simulink model "F15_NDI"  (R2020b)
settings: Solver=ode4  StartTime=0.0  StopTime=10  FixedStep=0.01  RelTol=1e-3
libraries: pid_lib x6
settings Model: Creator=chenglingquan  LastModifiedBy=chenglingquan

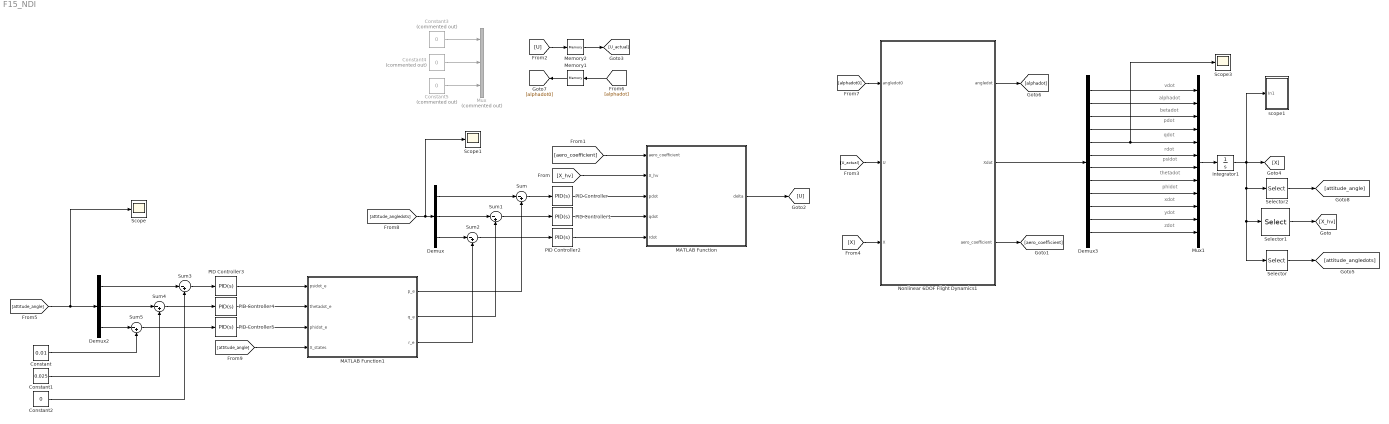
== system F15_NDI ==
  note: qdot
  note: thetadot
  note: zdot
  note: pdot
  note: ydot
  note: phidot
  note: xdot
  note: alphadot
  note: betadot
  note: psidot
  note: rdot
  note: vdot
  Constant : Constant  Value=0.01
  Constant1 : Constant  Value=0.025
  Constant2 : Constant  Value=0
  Constant3 : Constant  Commented=on  Value=0
  Constant4 : Constant  Commented=on  Value=0
  Constant5 : Constant  Commented=on  Value=0
  Demux : Demux  Outputs=3
  Demux2 : Demux  Outputs=3
  Demux3 : Demux  Outputs=12
  Integrator1 : Integrator  InitialCondition=[700,0.05,0,0,0,0,0,0,0,0,0,-6000]
  MATLAB Function : MATLAB Function  TreatAsAtomicUnit=on
  MATLAB Function1 : MATLAB Function  TreatAsAtomicUnit=on
  Memory1 : Memory  InitialCondition=[0,0]
  Memory2 : Memory  InitialCondition=[0,0,0]
  Mux : Mux  Commented=on  Inputs=3
  Mux1 : Mux  Inputs=12
  Nonlinear 6DOF Flight Dynamics1 : MATLAB Function  TreatAsAtomicUnit=on
  PID Controller : pid_lib/PID Controller  Controller=PID  Form=Parallel  TimeDomain=Continuous-time  UseExternalTs=off  SampleTime=-1  IntegratorMethod=Forward Euler  FilterMethod=Forward Euler  ControllerParametersSource=internal  P=50  I=1000  D=0  UseFilter=on  N=10000  TunerSelectOption=Transfer Function Based (PID Tuner App)  InitialConditionSource=internal  InitialConditionForIntegrator=0  InitialConditionForFilter=0  DifferentiatorICPrevScaledInput=0  ExternalReset=none  TrackingMode=off  Kt=1  LimitOutput=off  SatLimitsSource=internal  UpperSaturationLimit=inf  LowerSaturationLimit=-inf  LinearizeAsGain=on  AntiWindupMode=none  Kb=1  POutMin=[]  POutMax=[]  IOutMin=[]  IOutMax=[]  DOutMin=[]  DOutMax=[]  NOutMin=[]  NOutMax=[]  SumOutMin=[]  SumOutMax=[]  SaturationOutMin=[]  SaturationOutMax=[]  PParamMin=[]  PParamMax=[]  IParamMin=[]  IParamMax=[]  DParamMin=[]  DParamMax=[]  NParamMin=[]  NParamMax=[]  KbParamMin=[]  KbParamMax=[]  KtParamMin=[]  KtParamMax=[]  KbOutMin=[]  KbOutMax=[]  KtOutMin=[]  KtOutMax=[]  IntegratorOutMin=[]  IntegratorOutMax=[]  FilterOutMin=[]  FilterOutMax=[]  SumI1OutMin=[]  SumI1OutMax=[]  SumI2OutMin=[]  SumI2OutMax=[]  SumI3OutMin=[]  SumI3OutMax=[]  SumI4OutMin=[]  SumI4OutMax=[]  SumDOutMin=[]  SumDOutMax=[]  DifferentiatorOutMin=[]  DifferentiatorOutMax=[]  FilterDiffOutCoefMin=[]  FilterDiffOutCoefMax=[]  ReciprocalOutMin=[]  ReciprocalOutMax=[]  SumDenOutMin=[]  SumDenOutMax=[]  SumNumOutMin=[]  SumNumOutMax=[]  DivideOutMin=[]  DivideOutMax=[]  UdiffTsProdOutMin=[]  UdiffTsProdOutMax=[]  NTsProdOutMin=[]  NTsProdOutMax=[]  UintegralTsProdOutMin=[]  UintegralTsProdOutMax=[]  UngainTsProdOutMin=[]  UngainTsProdOutMax=[]  IntegratorContinuousStateAttributes=''  IntegratorStateMustResolveToSignalObject=off  IntegratorRTWStateStorageClass=Auto  FilterContinuousStateAttributes=''  FilterStateMustResolveToSignalObject=off  FilterRTWStateStorageClass=Auto  ParallelPVariant=InternalParameters  IdealPVariant=Disabled  IVariant=InternalParameters  DVariant=InternalParameters  IntegratorVariant=Continuous  SatVariant=Disabled  AWVariant=Passthrough  PCopyVariant=Disabled  TRVariant=Disabled  FdbkBlocksVariant=Forward  IdealPFdbkVariant=Disabled  SatFdbkVariant=Disabled  DerivativeFilterVariant=ContFilter  NVariant=InternalParameters  NCopyVariant=Disabled  FilterICVariant=InternalICsFilter  IntegratorICVariant=InternalICs  ExternalResetVariant=Disabled  TRSumVariant=Passthrough  SumFdbkVariant=Disabled  SumVariant=Sum_PID  TsampFilterVariant=InternalTs  TsampNgainVariant=Passthrough  TsampIntegralVariant=Passthrough  ExternalSaturationOutDataTypeStr=Inherit: Same as second input
  PID Controller1 : pid_lib/PID Controller  Controller=PID  Form=Parallel  TimeDomain=Continuous-time  UseExternalTs=off  SampleTime=-1  IntegratorMethod=Forward Euler  FilterMethod=Forward Euler  ControllerParametersSource=internal  P=20  I=100  D=0  UseFilter=on  N=500  TunerSelectOption=Transfer Function Based (PID Tuner App)  InitialConditionSource=internal  InitialConditionForIntegrator=0  InitialConditionForFilter=0  DifferentiatorICPrevScaledInput=0  ExternalReset=none  TrackingMode=off  Kt=1  LimitOutput=off  SatLimitsSource=internal  UpperSaturationLimit=inf  LowerSaturationLimit=-inf  LinearizeAsGain=on  AntiWindupMode=none  Kb=1  POutMin=[]  POutMax=[]  IOutMin=[]  IOutMax=[]  DOutMin=[]  DOutMax=[]  NOutMin=[]  NOutMax=[]  SumOutMin=[]  SumOutMax=[]  SaturationOutMin=[]  SaturationOutMax=[]  PParamMin=[]  PParamMax=[]  IParamMin=[]  IParamMax=[]  DParamMin=[]  DParamMax=[]  NParamMin=[]  NParamMax=[]  KbParamMin=[]  KbParamMax=[]  KtParamMin=[]  KtParamMax=[]  KbOutMin=[]  KbOutMax=[]  KtOutMin=[]  KtOutMax=[]  IntegratorOutMin=[]  IntegratorOutMax=[]  FilterOutMin=[]  FilterOutMax=[]  SumI1OutMin=[]  SumI1OutMax=[]  SumI2OutMin=[]  SumI2OutMax=[]  SumI3OutMin=[]  SumI3OutMax=[]  SumI4OutMin=[]  SumI4OutMax=[]  SumDOutMin=[]  SumDOutMax=[]  DifferentiatorOutMin=[]  DifferentiatorOutMax=[]  FilterDiffOutCoefMin=[]  FilterDiffOutCoefMax=[]  ReciprocalOutMin=[]  ReciprocalOutMax=[]  SumDenOutMin=[]  SumDenOutMax=[]  SumNumOutMin=[]  SumNumOutMax=[]  DivideOutMin=[]  DivideOutMax=[]  UdiffTsProdOutMin=[]  UdiffTsProdOutMax=[]  NTsProdOutMin=[]  NTsProdOutMax=[]  UintegralTsProdOutMin=[]  UintegralTsProdOutMax=[]  UngainTsProdOutMin=[]  UngainTsProdOutMax=[]  IntegratorContinuousStateAttributes=''  IntegratorStateMustResolveToSignalObject=off  IntegratorRTWStateStorageClass=Auto  FilterContinuousStateAttributes=''  FilterStateMustResolveToSignalObject=off  FilterRTWStateStorageClass=Auto  ParallelPVariant=InternalParameters  IdealPVariant=Disabled  IVariant=InternalParameters  DVariant=InternalParameters  IntegratorVariant=Continuous  SatVariant=Disabled  AWVariant=Passthrough  PCopyVariant=Disabled  TRVariant=Disabled  FdbkBlocksVariant=Forward  IdealPFdbkVariant=Disabled  SatFdbkVariant=Disabled  DerivativeFilterVariant=ContFilter  NVariant=InternalParameters  NCopyVariant=Disabled  FilterICVariant=InternalICsFilter  IntegratorICVariant=InternalICs  ExternalResetVariant=Disabled  TRSumVariant=Passthrough  SumFdbkVariant=Disabled  SumVariant=Sum_PID  TsampFilterVariant=InternalTs  TsampNgainVariant=Passthrough  TsampIntegralVariant=Passthrough  ExternalSaturationOutDataTypeStr=Inherit: Same as second input
  PID Controller2 : pid_lib/PID Controller  Controller=PID  Form=Parallel  TimeDomain=Continuous-time  UseExternalTs=off  SampleTime=-1  IntegratorMethod=Forward Euler  FilterMethod=Forward Euler  ControllerParametersSource=internal  P=20  I=100  D=0  UseFilter=on  N=500  TunerSelectOption=Transfer Function Based (PID Tuner App)  InitialConditionSource=internal  InitialConditionForIntegrator=0  InitialConditionForFilter=0  DifferentiatorICPrevScaledInput=0  ExternalReset=none  TrackingMode=off  Kt=1  LimitOutput=off  SatLimitsSource=internal  UpperSaturationLimit=inf  LowerSaturationLimit=-inf  LinearizeAsGain=on  AntiWindupMode=none  Kb=1  POutMin=[]  POutMax=[]  IOutMin=[]  IOutMax=[]  DOutMin=[]  DOutMax=[]  NOutMin=[]  NOutMax=[]  SumOutMin=[]  SumOutMax=[]  SaturationOutMin=[]  SaturationOutMax=[]  PParamMin=[]  PParamMax=[]  IParamMin=[]  IParamMax=[]  DParamMin=[]  DParamMax=[]  NParamMin=[]  NParamMax=[]  KbParamMin=[]  KbParamMax=[]  KtParamMin=[]  KtParamMax=[]  KbOutMin=[]  KbOutMax=[]  KtOutMin=[]  KtOutMax=[]  IntegratorOutMin=[]  IntegratorOutMax=[]  FilterOutMin=[]  FilterOutMax=[]  SumI1OutMin=[]  SumI1OutMax=[]  SumI2OutMin=[]  SumI2OutMax=[]  SumI3OutMin=[]  SumI3OutMax=[]  SumI4OutMin=[]  SumI4OutMax=[]  SumDOutMin=[]  SumDOutMax=[]  DifferentiatorOutMin=[]  DifferentiatorOutMax=[]  FilterDiffOutCoefMin=[]  FilterDiffOutCoefMax=[]  ReciprocalOutMin=[]  ReciprocalOutMax=[]  SumDenOutMin=[]  SumDenOutMax=[]  SumNumOutMin=[]  SumNumOutMax=[]  DivideOutMin=[]  DivideOutMax=[]  UdiffTsProdOutMin=[]  UdiffTsProdOutMax=[]  NTsProdOutMin=[]  NTsProdOutMax=[]  UintegralTsProdOutMin=[]  UintegralTsProdOutMax=[]  UngainTsProdOutMin=[]  UngainTsProdOutMax=[]  IntegratorContinuousStateAttributes=''  IntegratorStateMustResolveToSignalObject=off  IntegratorRTWStateStorageClass=Auto  FilterContinuousStateAttributes=''  FilterStateMustResolveToSignalObject=off  FilterRTWStateStorageClass=Auto  ParallelPVariant=InternalParameters  IdealPVariant=Disabled  IVariant=InternalParameters  DVariant=InternalParameters  IntegratorVariant=Continuous  SatVariant=Disabled  AWVariant=Passthrough  PCopyVariant=Disabled  TRVariant=Disabled  FdbkBlocksVariant=Forward  IdealPFdbkVariant=Disabled  SatFdbkVariant=Disabled  DerivativeFilterVariant=ContFilter  NVariant=InternalParameters  NCopyVariant=Disabled  FilterICVariant=InternalICsFilter  IntegratorICVariant=InternalICs  ExternalResetVariant=Disabled  TRSumVariant=Passthrough  SumFdbkVariant=Disabled  SumVariant=Sum_PID  TsampFilterVariant=InternalTs  TsampNgainVariant=Passthrough  TsampIntegralVariant=Passthrough  ExternalSaturationOutDataTypeStr=Inherit: Same as second input
  PID Controller3 : pid_lib/PID Controller  Controller=PID  Form=Parallel  TimeDomain=Continuous-time  UseExternalTs=off  SampleTime=-1  IntegratorMethod=Forward Euler  FilterMethod=Forward Euler  ControllerParametersSource=internal  P=10  I=25  D=0  UseFilter=on  N=10000  TunerSelectOption=Transfer Function Based (PID Tuner App)  InitialConditionSource=internal  InitialConditionForIntegrator=0  InitialConditionForFilter=0  DifferentiatorICPrevScaledInput=0  ExternalReset=none  TrackingMode=off  Kt=1  LimitOutput=off  SatLimitsSource=internal  UpperSaturationLimit=inf  LowerSaturationLimit=-inf  LinearizeAsGain=on  AntiWindupMode=none  Kb=1  POutMin=[]  POutMax=[]  IOutMin=[]  IOutMax=[]  DOutMin=[]  DOutMax=[]  NOutMin=[]  NOutMax=[]  SumOutMin=[]  SumOutMax=[]  SaturationOutMin=[]  SaturationOutMax=[]  PParamMin=[]  PParamMax=[]  IParamMin=[]  IParamMax=[]  DParamMin=[]  DParamMax=[]  NParamMin=[]  NParamMax=[]  KbParamMin=[]  KbParamMax=[]  KtParamMin=[]  KtParamMax=[]  KbOutMin=[]  KbOutMax=[]  KtOutMin=[]  KtOutMax=[]  IntegratorOutMin=[]  IntegratorOutMax=[]  FilterOutMin=[]  FilterOutMax=[]  SumI1OutMin=[]  SumI1OutMax=[]  SumI2OutMin=[]  SumI2OutMax=[]  SumI3OutMin=[]  SumI3OutMax=[]  SumI4OutMin=[]  SumI4OutMax=[]  SumDOutMin=[]  SumDOutMax=[]  DifferentiatorOutMin=[]  DifferentiatorOutMax=[]  FilterDiffOutCoefMin=[]  FilterDiffOutCoefMax=[]  ReciprocalOutMin=[]  ReciprocalOutMax=[]  SumDenOutMin=[]  SumDenOutMax=[]  SumNumOutMin=[]  SumNumOutMax=[]  DivideOutMin=[]  DivideOutMax=[]  UdiffTsProdOutMin=[]  UdiffTsProdOutMax=[]  NTsProdOutMin=[]  NTsProdOutMax=[]  UintegralTsProdOutMin=[]  UintegralTsProdOutMax=[]  UngainTsProdOutMin=[]  UngainTsProdOutMax=[]  IntegratorContinuousStateAttributes=''  IntegratorStateMustResolveToSignalObject=off  IntegratorRTWStateStorageClass=Auto  FilterContinuousStateAttributes=''  FilterStateMustResolveToSignalObject=off  FilterRTWStateStorageClass=Auto  ParallelPVariant=InternalParameters  IdealPVariant=Disabled  IVariant=InternalParameters  DVariant=InternalParameters  IntegratorVariant=Continuous  SatVariant=Disabled  AWVariant=Passthrough  PCopyVariant=Disabled  TRVariant=Disabled  FdbkBlocksVariant=Forward  IdealPFdbkVariant=Disabled  SatFdbkVariant=Disabled  DerivativeFilterVariant=ContFilter  NVariant=InternalParameters  NCopyVariant=Disabled  FilterICVariant=InternalICsFilter  IntegratorICVariant=InternalICs  ExternalResetVariant=Disabled  TRSumVariant=Passthrough  SumFdbkVariant=Disabled  SumVariant=Sum_PID  TsampFilterVariant=InternalTs  TsampNgainVariant=Passthrough  TsampIntegralVariant=Passthrough  ExternalSaturationOutDataTypeStr=Inherit: Same as second input
  PID Controller4 : pid_lib/PID Controller  Controller=PID  Form=Parallel  TimeDomain=Continuous-time  UseExternalTs=off  SampleTime=-1  IntegratorMethod=Forward Euler  FilterMethod=Forward Euler  ControllerParametersSource=internal  P=5  I=12  D=0  UseFilter=on  N=500  TunerSelectOption=Transfer Function Based (PID Tuner App)  InitialConditionSource=internal  InitialConditionForIntegrator=0  InitialConditionForFilter=0  DifferentiatorICPrevScaledInput=0  ExternalReset=none  TrackingMode=off  Kt=1  LimitOutput=off  SatLimitsSource=internal  UpperSaturationLimit=inf  LowerSaturationLimit=-inf  LinearizeAsGain=on  AntiWindupMode=none  Kb=1  POutMin=[]  POutMax=[]  IOutMin=[]  IOutMax=[]  DOutMin=[]  DOutMax=[]  NOutMin=[]  NOutMax=[]  SumOutMin=[]  SumOutMax=[]  SaturationOutMin=[]  SaturationOutMax=[]  PParamMin=[]  PParamMax=[]  IParamMin=[]  IParamMax=[]  DParamMin=[]  DParamMax=[]  NParamMin=[]  NParamMax=[]  KbParamMin=[]  KbParamMax=[]  KtParamMin=[]  KtParamMax=[]  KbOutMin=[]  KbOutMax=[]  KtOutMin=[]  KtOutMax=[]  IntegratorOutMin=[]  IntegratorOutMax=[]  FilterOutMin=[]  FilterOutMax=[]  SumI1OutMin=[]  SumI1OutMax=[]  SumI2OutMin=[]  SumI2OutMax=[]  SumI3OutMin=[]  SumI3OutMax=[]  SumI4OutMin=[]  SumI4OutMax=[]  SumDOutMin=[]  SumDOutMax=[]  DifferentiatorOutMin=[]  DifferentiatorOutMax=[]  FilterDiffOutCoefMin=[]  FilterDiffOutCoefMax=[]  ReciprocalOutMin=[]  ReciprocalOutMax=[]  SumDenOutMin=[]  SumDenOutMax=[]  SumNumOutMin=[]  SumNumOutMax=[]  DivideOutMin=[]  DivideOutMax=[]  UdiffTsProdOutMin=[]  UdiffTsProdOutMax=[]  NTsProdOutMin=[]  NTsProdOutMax=[]  UintegralTsProdOutMin=[]  UintegralTsProdOutMax=[]  UngainTsProdOutMin=[]  UngainTsProdOutMax=[]  IntegratorContinuousStateAttributes=''  IntegratorStateMustResolveToSignalObject=off  IntegratorRTWStateStorageClass=Auto  FilterContinuousStateAttributes=''  FilterStateMustResolveToSignalObject=off  FilterRTWStateStorageClass=Auto  ParallelPVariant=InternalParameters  IdealPVariant=Disabled  IVariant=InternalParameters  DVariant=InternalParameters  IntegratorVariant=Continuous  SatVariant=Disabled  AWVariant=Passthrough  PCopyVariant=Disabled  TRVariant=Disabled  FdbkBlocksVariant=Forward  IdealPFdbkVariant=Disabled  SatFdbkVariant=Disabled  DerivativeFilterVariant=ContFilter  NVariant=InternalParameters  NCopyVariant=Disabled  FilterICVariant=InternalICsFilter  IntegratorICVariant=InternalICs  ExternalResetVariant=Disabled  TRSumVariant=Passthrough  SumFdbkVariant=Disabled  SumVariant=Sum_PID  TsampFilterVariant=InternalTs  TsampNgainVariant=Passthrough  TsampIntegralVariant=Passthrough  ExternalSaturationOutDataTypeStr=Inherit: Same as second input
  PID Controller5 : pid_lib/PID Controller  Controller=PID  Form=Parallel  TimeDomain=Continuous-time  UseExternalTs=off  SampleTime=-1  IntegratorMethod=Forward Euler  FilterMethod=Forward Euler  ControllerParametersSource=internal  P=5  I=20  D=0  UseFilter=on  N=500  TunerSelectOption=Transfer Function Based (PID Tuner App)  InitialConditionSource=internal  InitialConditionForIntegrator=0  InitialConditionForFilter=0  DifferentiatorICPrevScaledInput=0  ExternalReset=none  TrackingMode=off  Kt=1  LimitOutput=off  SatLimitsSource=internal  UpperSaturationLimit=inf  LowerSaturationLimit=-inf  LinearizeAsGain=on  AntiWindupMode=none  Kb=1  POutMin=[]  POutMax=[]  IOutMin=[]  IOutMax=[]  DOutMin=[]  DOutMax=[]  NOutMin=[]  NOutMax=[]  SumOutMin=[]  SumOutMax=[]  SaturationOutMin=[]  SaturationOutMax=[]  PParamMin=[]  PParamMax=[]  IParamMin=[]  IParamMax=[]  DParamMin=[]  DParamMax=[]  NParamMin=[]  NParamMax=[]  KbParamMin=[]  KbParamMax=[]  KtParamMin=[]  KtParamMax=[]  KbOutMin=[]  KbOutMax=[]  KtOutMin=[]  KtOutMax=[]  IntegratorOutMin=[]  IntegratorOutMax=[]  FilterOutMin=[]  FilterOutMax=[]  SumI1OutMin=[]  SumI1OutMax=[]  SumI2OutMin=[]  SumI2OutMax=[]  SumI3OutMin=[]  SumI3OutMax=[]  SumI4OutMin=[]  SumI4OutMax=[]  SumDOutMin=[]  SumDOutMax=[]  DifferentiatorOutMin=[]  DifferentiatorOutMax=[]  FilterDiffOutCoefMin=[]  FilterDiffOutCoefMax=[]  ReciprocalOutMin=[]  ReciprocalOutMax=[]  SumDenOutMin=[]  SumDenOutMax=[]  SumNumOutMin=[]  SumNumOutMax=[]  DivideOutMin=[]  DivideOutMax=[]  UdiffTsProdOutMin=[]  UdiffTsProdOutMax=[]  NTsProdOutMin=[]  NTsProdOutMax=[]  UintegralTsProdOutMin=[]  UintegralTsProdOutMax=[]  UngainTsProdOutMin=[]  UngainTsProdOutMax=[]  IntegratorContinuousStateAttributes=''  IntegratorStateMustResolveToSignalObject=off  IntegratorRTWStateStorageClass=Auto  FilterContinuousStateAttributes=''  FilterStateMustResolveToSignalObject=off  FilterRTWStateStorageClass=Auto  ParallelPVariant=InternalParameters  IdealPVariant=Disabled  IVariant=InternalParameters  DVariant=InternalParameters  IntegratorVariant=Continuous  SatVariant=Disabled  AWVariant=Passthrough  PCopyVariant=Disabled  TRVariant=Disabled  FdbkBlocksVariant=Forward  IdealPFdbkVariant=Disabled  SatFdbkVariant=Disabled  DerivativeFilterVariant=ContFilter  NVariant=InternalParameters  NCopyVariant=Disabled  FilterICVariant=InternalICsFilter  IntegratorICVariant=InternalICs  ExternalResetVariant=Disabled  TRSumVariant=Passthrough  SumFdbkVariant=Disabled  SumVariant=Sum_PID  TsampFilterVariant=InternalTs  TsampNgainVariant=Passthrough  TsampIntegralVariant=Passthrough  ExternalSaturationOutDataTypeStr=Inherit: Same as second input
  Scope : Scope
  Scope1 : Scope
  Scope3 : Scope
  Selector : Selector  InputPortWidth=12  IndexOptions=Index vector (dialog)  Indices=[4 5 6]  OutputSizes=1
  Selector1 : Selector  InputPortWidth=12  IndexOptions=Index vector (dialog)  Indices=[2 3 4 5 6]  OutputSizes=1
  Selector2 : Selector  InputPortWidth=12  IndexOptions=Index vector (dialog)  Indices=[7 8 9]  OutputSizes=1
  Sum{,1..5} (6 alike) : Sum  Inputs=|-+
  scope1 : Subsystem
  wires:
  Demux3/1 -> Mux1/1
  Mux1/1 -> Integrator1/1
  Demux3/4 -> Mux1/4
  Demux3/7 -> Mux1/7
  Integrator1/1 -> [X], Selector2/1, Selector1/1, Selector/1, scope1/1(In1)
  Demux3/8 -> Mux1/8
  Demux3/3 -> Mux1/3
  Demux3/11 -> Mux1/11
  Demux3/5 -> Scope3/1, Mux1/5
  Demux3/6 -> Mux1/6
  Demux3/9 -> Mux1/9
  Demux3/12 -> Mux1/12
  Nonlinear 6DOF Flight Dynamics1/2(Xdot) -> Demux3/1
  Demux3/10 -> Mux1/10
  Demux3/2 -> Mux1/2
  Selector1/1 -> [X_hv]
  [X_hv] -> MATLAB Function/2(X_hv)
  Nonlinear 6DOF Flight Dynamics1/3(aero_coefficient) -> [aero_coefficient]
  [U] -> Memory2/1
  Memory2/1 -> [U_actual]
  [aero_coefficient] -> MATLAB Function/1(aero_coefficient)
  [X] -> Nonlinear 6DOF Flight Dynamics1/3(X)
  Nonlinear 6DOF Flight Dynamics1/1(angledot) -> [alphadot]
  [alphadot] -> Memory1/1
  Memory1/1 -> [alphadot0]
  [alphadot0] -> Nonlinear 6DOF Flight Dynamics1/1(angledot0)
  [attitude_angledots] -> Scope1/1, Demux/1
  Demux/1 -> Sum/1
  Demux/2 -> Sum1/1
  Demux/3 -> Sum2/1
  Sum/1 -> PID Controller/1
  Sum1/1 -> PID Controller1/1
  Sum2/1 -> PID Controller2/1
  Constant3/1 -> Mux/1
  Constant4/1 -> Mux/2
  Constant5/1 -> Mux/3
  [U_actual] -> Nonlinear 6DOF Flight Dynamics1/2(U)
  MATLAB Function/1(delta) -> [U]
  Selector/1 -> [attitude_angledots]
  PID Controller/1 -> MATLAB Function/3(pdot)
  PID Controller2/1 -> MATLAB Function/5(rdot)
  PID Controller1/1 -> MATLAB Function/4(qdot)
  Selector2/1 -> [attitude_angle]
  Demux2/2 -> Sum4/1
  Constant1/1 -> Sum4/2
  Constant/1 -> Sum5/2
  Sum5/1 -> PID Controller5/1
  Constant2/1 -> Sum3/2
  Sum3/1 -> PID Controller3/1
  Demux2/3 -> Sum5/1
  Sum4/1 -> PID Controller4/1
  Demux2/1 -> Sum3/1
  [attitude_angle] -> Scope/1, Demux2/1
  PID Controller3/1 -> MATLAB Function1/1(psidot_e)
  PID Controller4/1 -> MATLAB Function1/2(thetadot_e)
  PID Controller5/1 -> MATLAB Function1/3(phidot_e)
  [attitude_angle] -> MATLAB Function1/4(X_states)
  MATLAB Function1/1(p_e) -> Sum/2
  MATLAB Function1/2(q_e) -> Sum1/2
  MATLAB Function1/3(r_e) -> Sum2/2

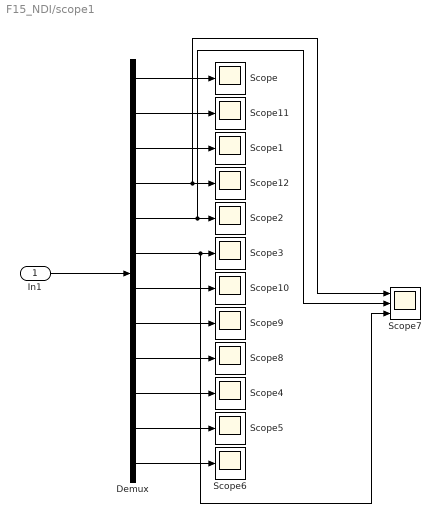
== system F15_NDI/scope1 ==
  In1 : Inport
  Demux : Demux  Outputs=12
  Scope{,1..6,8..12} (12 alike) : Scope
  Scope7 : Scope  NumInputPorts=3
  wires:
  Demux/7 -> Scope10/1
  Demux/4 -> Scope7/1, Scope12/1
  Demux/3 -> Scope1/1
  Demux/1 -> Scope/1
  Demux/8 -> Scope9/1
  Demux/9 -> Scope8/1
  Demux/5 -> Scope7/2, Scope2/1
  Demux/6 -> Scope7/3, Scope3/1
  Demux/2 -> Scope11/1
  In1/1 -> Demux/1
  Demux/10 -> Scope4/1
  Demux/11 -> Scope5/1
  Demux/12 -> Scope6/1

== matlab function F15_NDI/MATLAB Function1 ==
  data: psidot_e input; p_e output; thetadot_e input; phidot_e input; q_e output; r_e output; X_states input
function [p_e,q_e,r_e] = fcn(psidot_e,thetadot_e,phidot_e,X_states)
[psi,theta,phi] = deal(X_states(1),X_states(2),X_states(3));
G = [1 tan(theta)*sin(psi) tan(theta)*cos(psi);0 cos(psi) -sin(psi);0 sin(psi)/cos(theta) cos(psi)/cos(theta)];
angledot_e = inv(G)*[psidot_e;thetadot_e;phidot_e];
p_e = angledot_e(1);
q_e = angledot_e(2);
r_e = angledot_e(3);

== matlab function F15_NDI/MATLAB Function ==
  data: aero_coefficient input; delta output; X_hv input; pdot input; qdot input; rdot input
function delta  = fcn(aero_coefficient,X_hv,pdot,qdot,rdot)
%%

[alpha,beta,p,q,r] = deal(X_hv(1),X_hv(2),X_hv(3),X_hv(4),X_hv(5));
[C_lbeta,C_lda,C_lde,C_ldr,C_lr,C_lp,C_malpha,C_mda,C_mde,C_mdr,C_mq,C_nbeta,C_nda,C_nde,C_ndr,C_nr,C_np,C_malphadot,alphadot] = deal(aero_coefficient(1),...
    aero_coefficient(2),...
    aero_coefficient(3),...
    aero_coefficient(4),...
    aero_coefficient(5),...
    aero_coefficient(6),...
    aero_coefficient(7),...
    aero_coefficient(8),...
    aero_coefficient(9),...
    aero_coefficient(10),...
    aero_coefficient(11),...
    aero_coefficient(12),...
    aero_coefficient(13),...
    aero_coefficient(14),...
    aero_coefficient(15),...
    aero_coefficient(16),...
    aero_coefficient(17),...
    aero_coefficient(18),...
    aero_coefficient(19));
Ixx = 38915.25;
Iyy = 233864.41;
Izz = 254779.66;

control=[pdot;...
         qdot;...
         rdot];
%%
f_omega = [((Iyy-Izz)*q*r+(C_lbeta*beta+C_lp*p+C_lr*r))/Ixx;...
           ((Izz-Ixx)*p*r+(C_malpha*alpha+C_mq*q+C_malphadot*alphadot))/Iyy;...
           ((Ixx-Iyy)*p*q+(C_nbeta*beta+C_nr*r+C_np*p))/Izz];
G_omega = diag([1/Ixx 1/Iyy 1/Izz])*[C_lda C_lde C_ldr;C_mda C_mde C_mdr;C_nda C_nde C_ndr];
G_omega_inv=[(C_ndr*Ixx)/(C_lda*C_ndr - C_ldr*C_nda),0,-(C_ldr*Izz)/(C_lda*C_ndr - C_ldr*C_nda);...
             0,Iyy/C_mde,0;...
             -(C_nda*Ixx)/(C_lda*C_ndr - C_ldr*C_nda),0,(C_lda*Izz)/(C_lda*C_ndr - C_ldr*C_nda)];
%%
delta = G_omega_inv*(control-f_omega);

% u1= (C_ldr*C_nbeta*beta - C_lbeta*C_ndr*beta - C_lp*C_ndr*p + C_ldr*C_np*p - C_lr*C_ndr*r + C_ldr*C_nr*r + C_ndr*Ixx*pdot - C_ldr*Izz*rdot + C_ldr*Ixx*p*q - C_ldr*Iyy*p*q - C_ndr*Iyy*q*r + C_ndr*Izz*q*r)/(C_lda*C_ndr - C_ldr*C_nda);
% u2= -(C_malpha*alpha + C_malphadot*alphadot + C_mq*q - Iyy*qdot - Ixx*p*r + Izz*p*r)/C_mde;
% u3= -(C_lda*C_nbeta*beta - C_lbeta*C_nda*beta - C_lp*C_nda*p + C_lda*C_np*p - C_lr*C_nda*r + C_lda*C_nr*r + C_nda*Ixx*pdot - C_lda*Izz*rdot + C_lda*Ixx*p*q - C_lda*Iyy*p*q - C_nda*Iyy*q*r + C_nda*Izz*q*r)/(C_lda*C_ndr - C_ldr*C_nda)

== matlab function F15_NDI/Nonlinear 6DOF Flight Dynamics1 ==
  data: angledot0 input; U input; X input; angledot output; Xdot output; aero_coefficient output
function [angledot,Xdot,aero_coefficient] = fcn(angledot0,U,X)

%给各变量赋值
[alphadot,betadot]=deal(angledot0(1),angledot0(2));
[v,alpha,beta,p,q,r,psi,theta,phi,x,y,z] = deal(X(1),X(2),X(3),X(4),X(5),X(6),X(7),X(8),X(9),X(10),X(11),X(12));
[da,de,dr]=deal(U(1),U(2),U(3));

%基本参数
gamma=1.4;
R=287;
m=12700.59;%飞机空重
s=56.49; %机翼面积
b=13.05;%翼展
c=4.86;%平均气动弦长
g_inital=9.80665; %重力加速度
g=g_inital-v^2*cos(theta-alpha)/(6371001+z);%修正后的重力加速度
[rho,temp] = gas_wrt_height(-z);
Q=1/2*rho*v*v; %飞机动压
vel_a = sqrt(gamma * R * temp);
mach = v / vel_a;  %马赫数
T0=79178.35; %milthrust

%惯性矩、转动惯量及其衍生表达式
Ixx=38915.25;
Iyy=233864.41;
Izz=254779.66;
Ixy=0;
Ixz=0;%是否简化
Iyz=0;
c1=((Iyy-Izz)*Izz-Ixz*Ixz)/(Ixx*Izz - Ixz*Ixz);
c2=(Ixx-Iyy+Izz)*Ixz/(Ixx*Izz-Ixz*Ixz);
c3=Izz/(Ixx*Izz-Ixz*Ixz);
c4=Ixz/(Ixx*Izz-Ixz*Ixz);
c5=(Izz-Ixx)/Iyy;
c6=Ixz/Iyy;
c7=1/Iyy;
c8=(Ixx*(Ixx-Iyy)+Ixz*Ixz)/(Ixx*Izz-Ixz*Ixz);
c9=Ixx/(Ixx*Izz-Ixz*Ixz);

%气动力与气动力矩模块
datas = load('params.mat');  %由于部分气动力和力矩系数会随着飞行参数变化而变化，故需要根据现有数据插值得到，首先将用于差值的数据导入
%推力
[tmp1, tmp2] = meshgrid(datas.T_mach_altitude(2:end, 1), datas.T_mach_altitude(1, 2:end));
T = T0*interp2(tmp1, tmp2, datas.T_mach_altitude(2:end, 2:end)', mach, -z, 'spline');

%阻力D（需要插值获得的参数为C_Dalpha_alphamach，C_Di_alpha，C_Dbeta_alpha）
[tmp1, tmp2] = meshgrid(datas.C_Dalpha_alphamach(2:end, 1), datas.C_Dalpha_alphamach(1, 2:end));
C_Dalpha_alphamach = interp2(tmp1, tmp2, datas.C_Dalpha_alphamach(2:end, 2:end)', alpha, mach, 'spline');
C_Di_alpha = interp1(datas.C_Di_alpha(:, 1), datas.C_Di_alpha(:, 2), alpha, 'Linear', 'extrap');
C_Dbeta_alpha = interp1(datas.C_Dbeta_alpha(:, 1), datas.C_Dbeta_alpha(:, 2), alpha, 'Linear', 'extrap');

C_Dalpha=Q*s*C_Dalpha_alphamach;
C_Di=Q*s*C_Di_alpha;
C_Dbeta=Q*s*C_Dbeta_alpha;
C_Dde=0.048*Q*s;

D=C_Dalpha*alpha+C_Di+C_Dbeta*beta+C_Dde*de;

%侧力Y（需要插值获得的参数为C_Ybeta_alpha）
C_Ybeta_alpha=interp1(datas.C_Ybeta_alpha(:, 1), datas.C_Ybeta_alpha(:, 2), alpha, 'Linear', 'extrap');

C_Ybeta=Q*s*C_Ybeta_alpha;
C_Yda=Q*s*-0.0012;
C_Ydr=Q*s*0.3724;

Y=C_Ybeta*beta+C_Yda*da+C_Ydr*dr;

%升力L（需要插值获得的参数为C_Lalpha_alphamach）
[tmp1, tmp2] = meshgrid(datas.C_Lalpha_alphamach(2:end, 1), datas.C_Lalpha_alphamach(1, 2:end));
C_Lalpha_alphamach = interp2(tmp1, tmp2, datas.C_Lalpha_alphamach(2:end, 2:end)', alpha, mach, 'spline');

C_Lalpha=Q*s*C_Lalpha_alphamach;
C_Lde=Q*s*0.5730;
C_Lalphadot=Q*s*17.2232*c/(2*v);
C_Lq=Q*s*-17.2232*c/(2*v);

L=C_Lalpha*alpha+C_Lde*de+C_Lalphadot*alphadot+C_Lq*q;

%滚转力矩C_l（需要插值获得的参数为C_lbeta_alpha，C_lp_alpha，C_lda_alpha）

C_lbeta_alpha=interp1(datas.C_lbeta_alpha(:, 1), datas.C_lbeta_alpha(:, 2), alpha, 'Linear', 'extrap');
C_lp_alpha=interp1(datas.C_lp_alpha(:, 1), datas.C_lp_alpha(:, 2), alpha, 'Linear', 'extrap');
C_lda_alpha=interp1(datas.C_lda_alpha(:, 1), datas.C_lda_alpha(:, 2), alpha, 'Linear', 'extrap');

C_lbeta=Q*s*b*C_lbeta_alpha;
C_lp=Q*s*b*b/(2*v)*C_lp_alpha;
C_lr=Q*s*b*b/(2*v)*0.0001;
C_lda=Q*s*b*C_lda_alpha;
C_ldr=Q*s*b*0.0115;
C_lde=0;

C_l=C_lbeta*beta+C_lp*p+C_lr*r+C_lda*da+C_ldr*dr;

%俯仰力矩C_m（需要插值获得的参数为C_malpha_alpha）
C_malpha_alpha=interp1(datas.C_malpha_alpha(:, 1), datas.C_malpha_alpha(:, 2), alpha, 'Linear', 'extrap');

C_malpha=Q*s*c*C_malpha_alpha;
C_malphadot=-11.8870*Q*s*c*c/(2*v)*0;
C_mM=-0.0000*Q*s*c;
C_mq=-4.7000*Q*s*c*c/(2*v);
C_mde=-0.4580*Q*s*c;
C_mda=0;
C_mdr=0;

C_m=C_malpha*alpha+C_malphadot*alphadot+C_mq*q+C_mde*de;

%偏航力矩C_n（需要插值获得的参数为C_nbeta_alpha，C_np_alpha，C_ndr_alpha）
C_nbeta_alpha=interp1(datas.C_nbeta_alpha(:, 1), datas.C_nbeta_alpha(:, 2), alpha, 'Linear', 'extrap');
C_np_alpha=interp1(datas.C_np_alpha(:, 1), datas.C_np_alpha(:, 2), alpha, 'Linear', 'extrap');
C_ndr_alpha=interp1(datas.C_ndr_alpha(:, 1), datas.C_ndr_alpha(:, 2), alpha, 'Linear', 'extrap');

C_nbeta=C_nbeta_alpha*Q*s*b;
C_np=C_np_alpha*Q*s*b*b/(2*v);
C_nr=-0.4447*Q*s*b*b/(2*v);
C_nda=0.0022*Q*s*b;
C_ndr=C_ndr_alpha*Q*s*b;
C_nde=0;

C_n=C_nbeta*beta+C_np*p+C_nr*r+C_nda*da+C_ndr*dr;

%飞机速度v在机体坐标系下的分量
vx=v*cos(alpha)*cos(beta);
vy=v*sin(beta);
vz=v*sin(alpha)*cos(beta);

%空气动力A在机体坐标系下的分量
Xb=-D*cos(alpha)*cos(beta)-Y*cos(alpha)*sin(beta)+L*sin(alpha);
Yb=-D*sin(beta)+Y*cos(beta);
Zb=-D*sin(alpha)*cos(beta)-Y*sin(alpha)*sin(beta)-L*cos(alpha);

%体轴系下合外力的分量
Fx=T+Xb-m*g*sin(theta);
Fy=Yb+m*g*sin(psi)*cos(theta);
Fz=Zb+m*g*cos(psi)*cos(theta);

%体轴系质心动力学方程组

vdot=-((T+Xb)/m-g*sin(theta))*cos(alpha)*cos(beta)-(Yb/m+g*sin(psi)*cos(theta))*sin(beta)+(Zb/m-g*cos(psi)*cos(theta))*sin(alpha)*cos(beta);
alphadot=q+1/cos(beta)*((-(T+Xb)/(m*v)+g/v*sin(theta)-r*sin(beta))*sin(alpha)+(Zb/(m*v)+g/v*cos(psi)*cos(theta)-p*sin(beta))*cos(alpha));
betadot=-((Xb/(m*v)-g/v*sin(theta))*sin(beta)+r)*cos(alpha)+(Yb/(m*v)+g/v*sin(psi)*cos(theta))*cos(beta)+((-Zb/(m*v)-g/v*cos(psi)*cos(theta))*sin(beta)+p)*sin(alpha);
% gammadot=p*cos(alpha)*tan(beta)-q*(1-cos(psi))+r*(sin(alpha)*tan(beta)-sin(psi))+(Fx*sin(alpha)-Fz*cos(alpha))/(m*v);

%体轴系绕质心运动学方程组
pdot = (C_l+(Iyy-Izz)*q*r)/Ixx;
qdot = (C_m+(Izz-Ixx)*p*r)/Iyy;
rdot = (C_n+(Ixx-Iyy)*p*q)/Izz;

%将p,q,r从机体坐标系转换到地理坐标系,得到欧拉角的计算方程式
psidot = p+tan(theta)*(q*sin(psi)+r*cos(psi));
thetadot = q*cos(psi)-r*sin(psi);
phidot = 1/cos(theta)*(q*sin(psi)+r*cos(psi));

%飞机运动位置
%将飞机质心速度V在机体坐标系上的分量vx,vy,vz转换到地面坐标系上
xdot =  cos(theta)*cos(phi)*vx+(cos(phi)*sin(psi)*sin(theta) - cos(psi)*sin(phi))*vy+(sin(psi)*sin(phi) + cos(psi)*cos(phi)*sin(theta))*vz;
ydot =  cos(theta)*sin(phi)*vx+(cos(psi)*cos(phi) + sin(psi)*sin(theta)*sin(phi))*vy+(cos(psi)*sin(theta)*sin(phi) - cos(phi)*sin(psi))*vz;
zdot =  -sin(theta)*vx+cos(theta)*sin(psi)*vy+cos(psi)*cos(theta)*vz;


%%
Xdot=[vdot,alphadot,betadot,pdot,qdot,rdot,psidot,thetadot,phidot,xdot,ydot,zdot];
angledot=[alphadot,betadot];
%aerodynamic coefficient
aero_coefficient=[C_lbeta,C_lda,C_lde,C_ldr,C_lr,C_lp,C_malpha,C_mda,C_mde,C_mdr,C_mq,C_nbeta,C_nda,C_nde,C_ndr,C_nr,C_np,beta,alpha,C_malphadot,alphadot];
% Edot=[e0dot,e1dot,e2dot,e3dot];
